simulink model "Brk_VD"  (R2016b)
settings: configuration reference "CodeGenConfigSet" (kept outside this file)
values from neighbouring files (symbols this model uses):
  Brk_tiPlaDebDef_C = Calibration.Parameter    [init_Brk_VD.m]
  Brk_tiPlaDebOk_C = Calibration.Parameter    [init_Brk_VD.m]
undefined symbols (not defined in the file or in its folder): Brk_VD_DT
settings Model: Creator=lenovo  LastModifiedBy=lenovo
settings ConfigSetRef: SourceLocation=Base Workspace

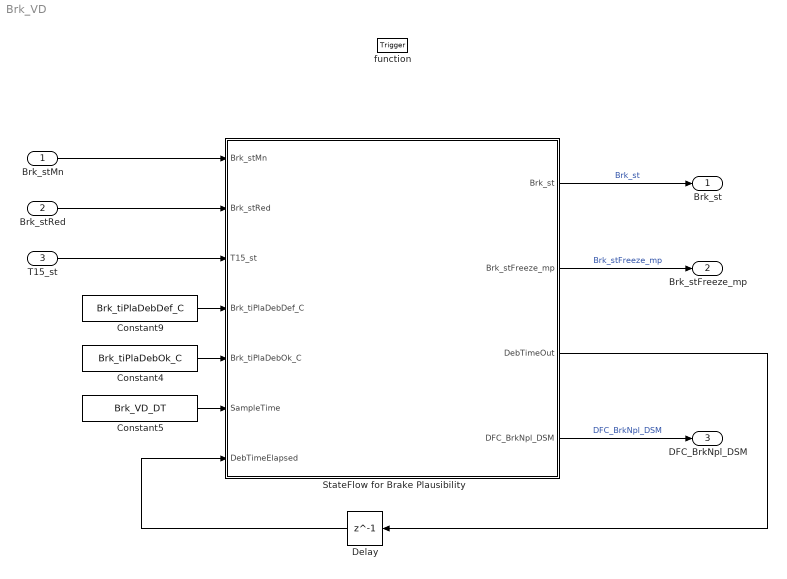
== system Brk_VD ==
  Brk_stMn : Inport  Description=Status of the main brake  OutMin=0  OutMax=1  OutDataTypeStr=boolean
  Brk_stRed : Inport  Description=Status of the redundant break  Port=2  OutMin=0  OutMax=1  OutDataTypeStr=boolean
  T15_st : Inport  Description=Terminal 15 status after debouncing  Port=3  OutDataTypeStr=Enum: Switch_conv
  function : TriggerPort  TriggerType=function-call  VariantControl=Variant
  Constant4 : Constant  Value=Brk_tiPlaDebOk_C
  Constant5 : Constant  Value=Brk_VD_DT  OutDataTypeStr=Inherit: Inherit via back propagation
  Constant9 : Constant  Value=Brk_tiPlaDebDef_C
  Delay : Delay  DelayLength=1  InitialCondition=0
  StateFlow for Brake Plausibility : Stateflow chart
  Brk_st : Outport  Description=Brake switch state  OutMin=0  OutMax=255  OutDataTypeStr=State_uint8
  Brk_stFreeze_mp : Outport  Description=Measuring Point to indicate whether the brake plausibility state machine is in Neutral State  Port=2  OutMin=0  OutMax=1  OutDataTypeStr=boolean
  DFC_BrkNpl_DSM : Outport  Description="state of error\"DFC_BrkNpl\""  Port=3  OutMin=0  OutMax=1  OutDataTypeStr=boolean
  wires:
  StateFlow for Brake Plausibility/4(DFC_BrkNpl_DSM) -> DFC_BrkNpl_DSM/1  "DFC_BrkNpl_DSM"
  StateFlow for Brake Plausibility/2(Brk_stFreeze_mp) -> Brk_stFreeze_mp/1  "Brk_stFreeze_mp"
  Constant5/1 -> StateFlow for Brake Plausibility/6(SampleTime)
  Constant4/1 -> StateFlow for Brake Plausibility/5(Brk_tiPlaDebOk_C)
  Constant9/1 -> StateFlow for Brake Plausibility/4(Brk_tiPlaDebDef_C)
  Delay/1 -> StateFlow for Brake Plausibility/7(DebTimeElapsed)
  StateFlow for Brake Plausibility/3(DebTimeOut) -> Delay/1
  StateFlow for Brake Plausibility/1(Brk_st) -> Brk_st/1  "Brk_st"
  T15_st/1 -> StateFlow for Brake Plausibility/3(T15_st)
  Brk_stRed/1 -> StateFlow for Brake Plausibility/2(Brk_stRed)
  Brk_stMn/1 -> StateFlow for Brake Plausibility/1(Brk_stMn)

== stateflow chart Brk_VD/StateFlow for Brake Plausibility ==
  settings: sampleTime=0.01
  note: %为State3添加了T15=0的自循环
  state State1
    entry:	DebTimeOut = 0;
    DFC_BrkNpl_DSM = 0;
  state State5
    entry: Brk_st = 0x00;
    Brk_stFreeze_mp = 1;
  state State4
    entry: Brk_st = 0x03;
  state State2
    entry:Brk_st = 0x01;
  state State3
    entry:   Brk_st = 0x01;
    DFC_BrkNpl_DSM =1;
  (default) -> State1
  State1 -> State1 [order 2] : [(Brk_stMn ==0x00)&&...
      | (Brk_stRed ==0x00)]{Brk_st = 0x00;}
  State1 -> State1 [order 3] : [(Brk_stMn ==0x01)&&...
      | (Brk_stRed ==0x01)]{Brk_st = 0x03;}
  State1 -> State2 [order 1] : [Brk_stMn ~= Brk_stRed]
  State4 -> State1 [order 2] : [(Brk_stMn==0x01)&&(Brk_stRed==0x01)&&...
      | (DebTimeElapsed>=Brk_tiPlaDebOk_C)]
  State5 -> State1 [order 1] : [((Brk_stMn == 0x01)&&(Brk_stRed==0x01))||...
      | (T15_st==0x00)]{Brk_stFreeze_mp = 0}
  State2 -> State1 [order 1] : [((Brk_stMn ==0x01)&&(Brk_stRed==0x01))||...
      | (T15_st == 0x00)]
  State4 -> State4 [order 3] : [(Brk_stMn==0x01)&&(Brk_stRed==0x01)&&...
      | (DebTimeElapsed<Brk_tiPlaDebOk_C)]{DebTimeOut+=SampleTime;}
  State2 -> State5 [order 2] : [(Brk_stMn == 0x00)&&(Brk_stRed==0x00)]...
  State2 -> State2 [order 4] : [(Brk_stMn ~= Brk_stRed)&&...
      | (DebTimeElapsed<Brk_tiPlaDebDef_C)]{DebTimeOut += SampleTime;}
  State3 -> State4 [order 2] : [(Brk_stMn==0x01)&&(Brk_stRed==0x01)]...
      | {DebTimeOut=0x00;}
  State4 -> State3 [order 1] : [(Brk_stMn==0x00) ||(Brk_stRed==0x00)||(T15_st==0x00)]
  State5 -> State5 [order 3] : [(Brk_stMn == 0x00)&&(Brk_stRed==0x00)]
  State5 -> State2 [order 2] : [Brk_stMn ~= Brk_stRed]{Brk_stFreeze_mp = 0}
  State2 -> State3 [order 3] : [(Brk_stMn ~= Brk_stRed)&&...
      | (DebTimeElapsed>=Brk_tiPlaDebDef_C)]
  State3 -> State3 [order 1] : [T15_st==0x00]
  State3 -> State3 [order 3] : [(Brk_stMn==0x00) ||(Brk_stRed==0x00)]
  data: Brk_st output; Brk_stFreeze_mp output; Brk_stMn input; Brk_stRed input; T15_st input; Brk_tiPlaDebDef_C input; Brk_tiPlaDebOk_C input; SampleTime input uint16 =1; DebTimeOut output uint16; DebTimeElapsed input; DFC_BrkNpl_DSM output boolean
